simulink model "InvLamp"  (Simulink 7.0)
settings: Solver=ode45  SolverMode=SingleTasking  StartTime=0.0  StopTime=10.0  RelTol=1e-3  AbsTol=1e-6
settings Model: Creator=abbas  LastModifiedBy=abbas
settings DataIOCC: LimitDataPoints=off
settings OptimizationCC: BlockReduction=off  BooleanDataType=off  InlineInvariantSignals=on
settings DebuggingCC: SaveWithParameterizedLinksMsg=none  SignalResolutionControl=TryResolveAllWithWarning  SolverPrmCheckMsg=none  MultiTaskDSMMsg=warning  MultiTaskCondExecSysMsg=none  StrictBusMsg=None
settings HardwareCC: TargetUnknown=on
settings RTWCC: IncludeERTFirstTime=on
settings GRTTargetCC: TargetFcnLib=ansi_tfl_tmw.mat  ModelReferenceCompliant=off  CompOptLevelCompliant=off  MatFileLogging=off

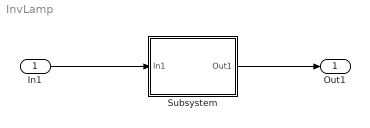
== system InvLamp ==
  In1 : Inport  OutDataType=sfix(16)  OutScaling=2^0
  Subsystem : Subsystem
  Out1 : Outport  OutDataType=sfix(16)  OutScaling=2^0
  wires:
  In1/1 -> Subsystem/1(In1)
  Subsystem/1(Out1) -> Out1/1

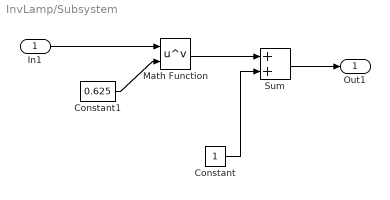
== system InvLamp/Subsystem ==
  In1 : Inport  OutDataType=sfix(16)  OutScaling=2^0
  Constant : Constant  OutDataType=sfix(16)  OutScaling=2^0
  Constant1 : Constant  Value=0.625  OutDataType=sfix(16)  OutScaling=2^0
  Math Function : Math  Operator=pow  OutDataType=sfix(16)  OutScaling=2^0  SaturateOnIntegerOverflow=on
  Sum : Sum  OutDataType=sfix(16)  OutScaling=2^0  SaturateOnIntegerOverflow=on  InputSameDT=on
  Out1 : Outport  OutDataType=sfix(16)  OutScaling=2^0
  wires:
  Constant1/1 -> Math Function/2
  Sum/1 -> Out1/1
  Constant/1 -> Sum/2
  In1/1 -> Math Function/1
  Math Function/1 -> Sum/1
